simulink library "headingSetpointCalculation_cl"  (R2018a)
settings: Solver=VariableStepAuto  StartTime=0.0  StopTime=10.0  RelTol=1e-3
libraries: flatlandHeading_ul x1, offsetLeadDistance_ul x1, pathPosition_ul x1, pathProjection_ul x1
settings Model: Creator=mcobb  LastModifiedBy=mcobb

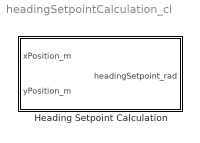
== system headingSetpointCalculation_cl ==
  Heading Setpoint Calculation : Subsystem

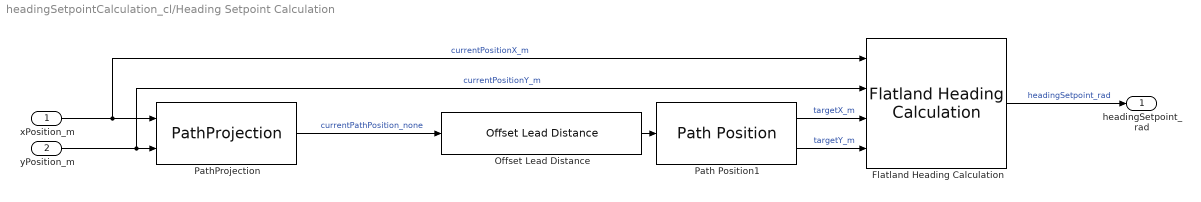
== system headingSetpointCalculation_cl/Heading Setpoint Calculation ==
  xPosition_m : Inport
  yPosition_m : Inport  Port=2
  Flatland Heading Calculation : flatlandHeading_ul/Flatland Heading Calculation
  Offset Lead Distance : offsetLeadDistance_ul/Offset Lead Distance
  Path Position1 : pathPosition_ul/Path Position
  PathProjection : pathProjection_ul/PathProjection
  headingSetpoint_rad : Outport
  wires:
  Offset Lead Distance/1 -> Path Position1/1
  Flatland Heading Calculation/1 -> headingSetpoint_rad/1  "headingSetpoint_rad"
  PathProjection/1 -> Offset Lead Distance/1  "currentPathPosition_none"
  Path Position1/1 -> Flatland Heading Calculation/3  "targetX_m"
  Path Position1/2 -> Flatland Heading Calculation/4  "targetY_m"
  xPosition_m/1 -> Flatland Heading Calculation/1, PathProjection/1  "currentPositionX_m"
  yPosition_m/1 -> Flatland Heading Calculation/2, PathProjection/2  "currentPositionY_m"
